simulink model "KugleSim_VelocityLQR"  (R2018a)
settings: Solver=VariableStepAuto  StartTime=0.0  StopTime=35  FixedStep=1e-3  MaxStep=1e-2  RelTol=1e-5
PreLoadFcn:
  | modelDir = fileparts(get_param(bdroot, 'FileName'));
  | addpath(fullfile(modelDir,'../Parameters'));
  | addpath(fullfile(modelDir,'subsystems'));
  | 
  | Parameters_General
  | Parameters_Simulation
  | Parameters_Controllers
InitFcn:
  | Parameters_General
  | Parameters_Simulation
  | Parameters_Controllers
StopFcn:
  | StructurizeLoggedData
values from neighbouring files (symbols this model uses):
  Ts = 1/200    (= 0.005)    [Parameters_Controller.m]
libraries: simulink x1
settings Model: Creator=Thomas  LastModifiedBy=Thomas
settings DebuggingCC: UniqueDataStoreMsg=error
settings HardwareCC: ProdBitPerPointer=32  ProdBitPerSizeT=32  ProdBitPerPtrDiffT=32  ProdLargestAtomicInteger=Long  ProdLargestAtomicFloat=Double  ProdWordSize=32  ProdHWDeviceType=ARM Compatible->ARM Cortex
settings ModelReferenceCC: ModelReferenceNumInstancesAllowed=Zero
settings RTWCC: GenCodeOnly=on  Toolchain=GNU Tools for ARM Embedded Processors
settings GRTTargetCC: TargetLangStandard=C89/C90 (ANSI)  CodeReplacementLibrary=ARM Cortex-M (CMSIS)

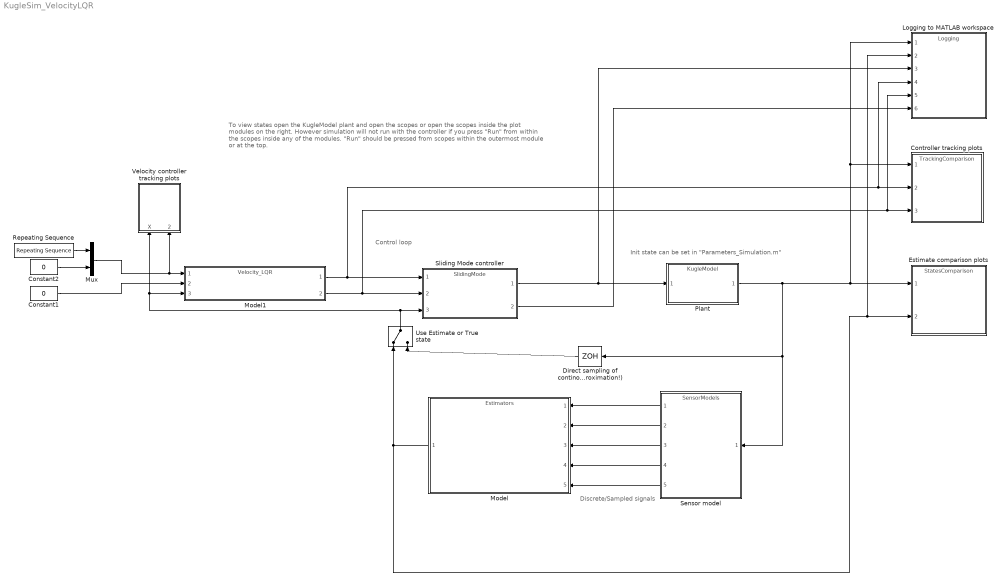
== system KugleSim_VelocityLQR ==
  note: Control loop
  note: Discrete/Sampled signals
  note: Init state can be set in "Parameters_Simulation.m"
  note: To view states open the KugleModel plant and open the scopes or open the scopes inside the plot modules on the right.
      | However simulation will not run with the controller if you press "Run" from within the scopes inside any of the modules.
      | "Run" should be pressed from scopes within the outermost module or at the top.
  Constant1 : Constant  Value=0  SampleTime=Ts
  Constant2 : Constant  Value=0  SampleTime=Ts
  Controller tracking plots : ModelReference  ModelNameDialog=TrackingComparison  SimulationMode=Normal  ModelReferenceVersion=1.13
  Direct sampling of continous states (simple/approximation!) : ZeroOrderHold  SampleTime=Ts
  Estimate comparison plots : ModelReference  ModelNameDialog=StatesComparison  SimulationMode=Normal  ModelReferenceVersion=1.9
  Logging to MATLAB workspace : ModelReference  ModelNameDialog=Logging  SimulationMode=Normal  ModelReferenceVersion=1.12
  Model : ModelReference  ModelNameDialog=Estimators  SimulationMode=Normal  ModelReferenceVersion=1.12
  Model1 : ModelReference  ModelNameDialog=Velocity_LQR  SimulationMode=Normal  ModelReferenceVersion=1.67
  Mux : Mux  Inputs=2
  Plant : ModelReference  ModelNameDialog=KugleModel  SimulationMode=Normal  ModelReferenceVersion=1.2094
  Repeating Sequence : simulink/Sources/Repeating Sequence  rep_seq_t=[0 8 10 15 17 22 24 29 31]  rep_seq_y=[0 0 1 1 0 0 -1 -1 0]
  Sensor model : ModelReference  ModelNameDialog=SensorModels  SimulationMode=Normal  ModelReferenceVersion=1.18
  Sliding Mode controller : ModelReference  ModelNameDialog=SlidingMode  SimulationMode=Normal  ModelReferenceVersion=1.48
  Use Estimate or True state : ManualSwitch
  Velocity controller tracking plots : Subsystem
  wires:
  Direct sampling of continous states (simple/approximation!)/1 -> Use Estimate or True state/2
  Plant/1 -> Sensor model/1, Direct sampling of continous states (simple/approximation!)/1, Logging to MATLAB workspace/1, Controller tracking plots/1, Estimate comparison plots/1
  Model1/2 -> Logging to MATLAB workspace/5, Controller tracking plots/3, Sliding Mode controller/2
  Sliding Mode controller/1 -> Logging to MATLAB workspace/3, Plant/1
  Use Estimate or True state/1 -> Sliding Mode controller/3, Model1/3, Velocity controller tracking plots/1(X)
  Sensor model/5 -> Model/5
  Sensor model/4 -> Model/4
  Sensor model/2 -> Model/2
  Sensor model/3 -> Model/3
  Sensor model/1 -> Model/1
  Model/1 -> Use Estimate or True state/1, Logging to MATLAB workspace/2, Estimate comparison plots/2
  Sliding Mode controller/2 -> Logging to MATLAB workspace/6
  Model1/1 -> Logging to MATLAB workspace/4, Controller tracking plots/2, Sliding Mode controller/1
  Mux/1 -> Model1/1, Velocity controller tracking plots/2(v_ref_inertial)
  Constant1/1 -> Model1/2
  Repeating Sequence/1 -> Mux/1
  Constant2/1 -> Mux/2

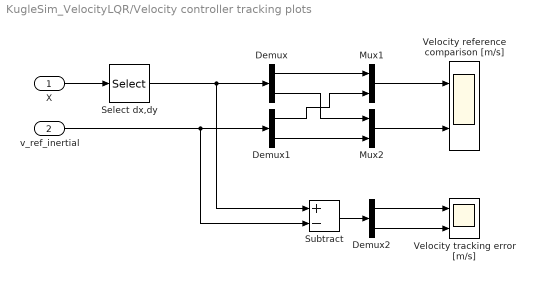
== system KugleSim_VelocityLQR/Velocity controller tracking plots ==
  X : Inport
  v_ref_inertial : Inport  Port=2
  Demux : Demux  Outputs=2
  Demux1 : Demux  Outputs=2
  Demux2 : Demux  Outputs=2
  Mux1 : Mux  Inputs=2
  Mux2 : Mux  Inputs=2
  Select dx,dy : Selector  InputPortWidth=12  IndexOptions=Index vector (dialog)  Indices=[7,8]  OutputSizes=1
  Subtract : Sum  Inputs=+-
  Velocity reference comparison [m/s] : Scope  NumInputPorts=2
  Velocity tracking error [m/s] : Scope  NumInputPorts=2
  wires:
  X/1 -> Select dx,dy/1
  Demux/1 -> Mux1/1
  Demux1/2 -> Mux2/2
  Mux1/1 -> Velocity reference comparison [m/s]/1
  Demux/2 -> Mux2/1
  v_ref_inertial/1 -> Subtract/2, Demux1/1
  Select dx,dy/1 -> Subtract/1, Demux/1
  Mux2/1 -> Velocity reference comparison [m/s]/2
  Demux1/1 -> Mux1/2
  Demux2/1 -> Velocity tracking error [m/s]/1
  Demux2/2 -> Velocity tracking error [m/s]/2
  Subtract/1 -> Demux2/1
